simulink model "nieLiniowyModelWachadlaOdwruconego"  (R2014a)
settings: Solver=ode45  SolverMode=SingleTasking  StartTime=0.0  StopTime=100  MaxStep=0.1  MinStep=0.001  RelTol=1e-5
values from neighbouring files (symbols this model uses):
  K0 = lqr(A0,B0,Q0,R0)    [WyznaczanieParametrow.m]
  K120 = lqr(A120,B120,Q120,R120)    [WyznaczanieParametrow.m]
  K150 = acker(A150,B150,[0 3 0 0])    [WyznaczanieParametrow.m]
  K30 = lqr(A30,B30,Q30,R30)    [WyznaczanieParametrow.m]
  K90 = lqr(A90,B90,Q90,R90)    [WyznaczanieParametrow.m]
undefined symbols (not defined in the file or in its folder): K180
libraries: fuzblock x1
settings Model: CovMetricSettings=dwe  CovHtmlReporting=off  covSaveCumulativeToWorkspaceVar=off  CovSaveSingleToWorkspaceVar=off  CovExternalEMLEnable=on  CovSFcnEnable=on  Creator=Szwank  LastModifiedBy=Szwank
settings DataIOCC: LimitDataPoints=off  SaveFormat=StructureWithTime
settings DebuggingCC: MergeDetectMultiDrivingBlocksExec=error  SolverPrmCheckMsg=none  FrameProcessingCompatibilityMsg=error  SFUnexpectedBacktrackingDiag=error  SFNoUnconditionalDefaultTransitionDiag=error
settings HardwareCC: ProdBitPerPointer=64  ProdLargestAtomicFloat=Float  ProdIntDivRoundTo=Zero  ProdEndianess=LittleEndian  ProdHWDeviceType=Specified
settings ModelReferenceCC: PropagateSignalLabelsOutOfModel=on
settings GRTTargetCC: TargetLangStandard=C99 (ISO)  GeneratePreprocessorConditionals=Use local settings

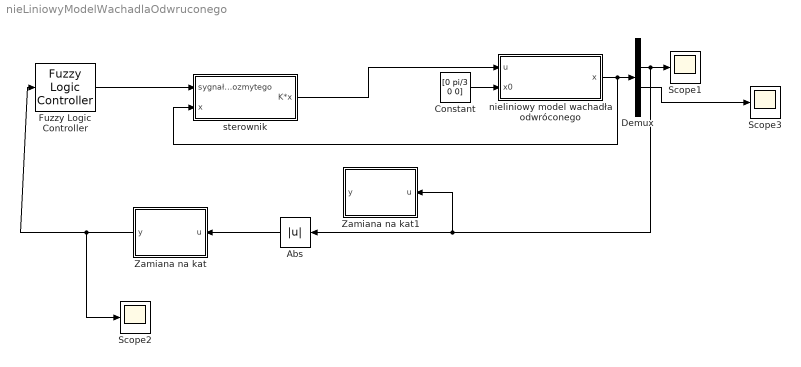
== system nieLiniowyModelWachadlaOdwruconego ==
  " nieliniowy model wachadła odwróconego" : Subsystem
  Abs : Abs
  Constant : Constant  Value=[0 pi/3 0 0]
  Demux : Demux
  Fuzzy Logic Controller : fuzblock/Fuzzy Logic  Controller  fis='modelRozmyty.fis'
  Scope1 : Scope
      settings: TimeRange=auto  MaxDataPoints=5000  SaveToWorkspace=off  YMin=-5.59281  YMax=1.78498  SampleTime=-1
  Scope2 : Scope
      settings: TimeRange=auto  MaxDataPoints=5000  SaveToWorkspace=off  YMin=-22.49983  YMax=202.49843  SampleTime=-1
  Scope3 : Scope
      settings: TimeRange=auto  MaxDataPoints=5000  SaveToWorkspace=off  SaveName=ScopeData3  YMin=-0.00269  YMax=0.0027  SampleTime=-1
  Zamiana na kat : MATLAB Function  TreatAsAtomicUnit=on
      settings: PermitHierarchicalResolution=ParametersOnly
  Zamiana na kat1 : MATLAB Function  TreatAsAtomicUnit=on
      settings: PermitHierarchicalResolution=ParametersOnly
  sterownik : Subsystem
  wires:
  Abs/1 -> Zamiana na kat/1(u)
  Zamiana na kat/1(y) -> Scope2/1, Fuzzy Logic Controller/1
  Constant/1 -> " nieliniowy model wachadła odwróconego"/2(x0)
  Demux/2 -> Zamiana na kat1/1(u), Abs/1, Scope1/1
  " nieliniowy model wachadła odwróconego"/1(x) -> sterownik/2("x "), Demux/1
  Fuzzy Logic Controller/1 -> sterownik/1(sygnał z regulatora rozmytego)
  sterownik/1(K*x) -> " nieliniowy model wachadła odwróconego"/1(u)
  Demux/3 -> Scope3/1

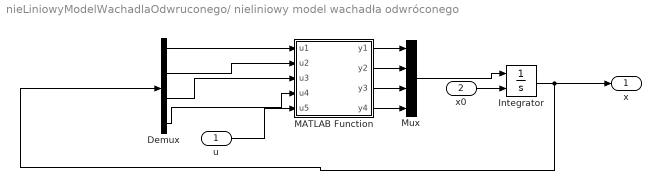
== system nieLiniowyModelWachadlaOdwruconego/ nieliniowy model wachadła odwróconego ==
  u : Inport
  x0 : Inport  Port=2
  Demux : Demux
  Integrator : Integrator  InitialConditionSource=external  InitialCondition=[0 pi/6 0 0]
  MATLAB Function : MATLAB Function  TreatAsAtomicUnit=on
      settings: PermitHierarchicalResolution=ParametersOnly
  Mux : Mux
  x : Outport
  wires:
  Mux/1 -> Integrator/1
  Demux/1 -> MATLAB Function/1(u1)
  MATLAB Function/2(y2) -> Mux/2
  Demux/4 -> MATLAB Function/4(u4)
  MATLAB Function/4(y4) -> Mux/4
  Integrator/1 -> x/1, Demux/1
  MATLAB Function/1(y1) -> Mux/1
  Demux/3 -> MATLAB Function/3(u3)
  MATLAB Function/3(y3) -> Mux/3
  Demux/2 -> MATLAB Function/2(u2)
  u/1 -> MATLAB Function/5(u5)
  x0/1 -> Integrator/2

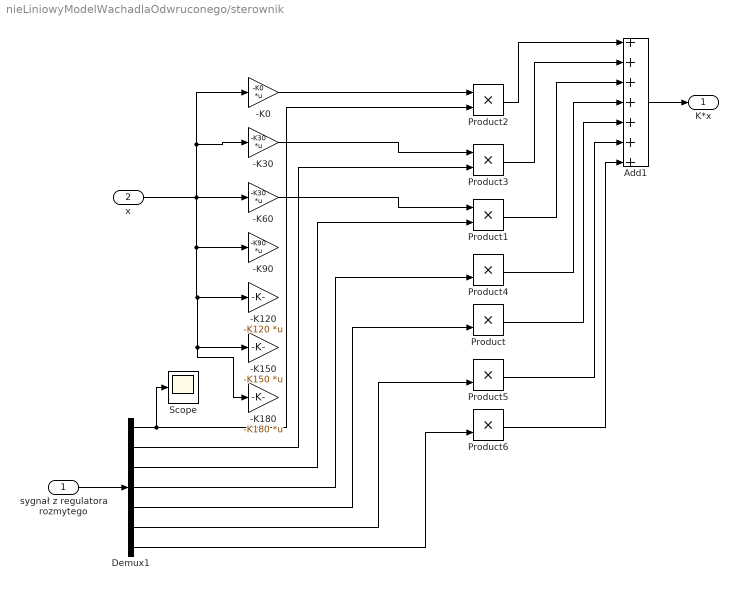
== system nieLiniowyModelWachadlaOdwruconego/sterownik ==
  sygnał z regulatora rozmytego : Inport
  "x " : Inport  Port=2
  -K0 : Gain  Gain=-K0  Multiplication=Matrix(K*u)
  "-K120 " : Gain  Gain=-K120  Multiplication=Matrix(K*u)
  "-K150 " : Gain  Gain=-K150  Multiplication=Matrix(K*u)
  -K180 : Gain  Gain=-K180  Multiplication=Matrix(K*u)
  -K30 : Gain  Gain=-K30  Multiplication=Matrix(K*u)
  -K60 : Gain  Gain=-K30  Multiplication=Matrix(K*u)
  -K90 : Gain  Gain=-K90  Multiplication=Matrix(K*u)
  Add1 : Sum  Inputs=+++++++
  Demux1 : Demux  Outputs=7
  Product{,1..6} (7 alike) : Product
  Scope : Scope
      settings: TimeRange=auto  MaxDataPoints=5000  SaveToWorkspace=off  SaveName=ScopeData2  YMin=-0.01968  YMax=1.02314  SampleTime=-1
  K*x : Outport
  wires:
  -K0/1 -> Product2/1
  sygnał z regulatora rozmytego/1 -> Demux1/1
  -K30/1 -> Product3/1
  Product3/1 -> Add1/2
  Demux1/1 -> Scope/1, Product2/2
  Product2/1 -> Add1/1
  Demux1/2 -> Product3/2
  "x "/1 -> -K180/1, "-K150 "/1, "-K120 "/1, -K90/1, -K60/1, -K30/1, -K0/1
  Add1/1 -> K*x/1
  Product1/1 -> Add1/3
  -K60/1 -> Product1/1
  Demux1/3 -> Product1/2
  Demux1/4 -> Product4/2
  Product4/1 -> Add1/4
  Demux1/5 -> Product/2
  Demux1/6 -> Product5/2
  Demux1/7 -> Product6/2
  Product/1 -> Add1/5
  Product5/1 -> Add1/6
  Product6/1 -> Add1/7

== matlab function nieLiniowyModelWachadlaOdwruconego/ nieliniowy model wachadła odwróconego/MATLAB Function ==
  data: u1 input; y1 output; u2 input; u3 input; u4 input; u5 input; y2 output; y3 output; y4 output
function [y1,y2,y3,y4] = fcn(u1,u2,u3,u4,u5)
%Dane obiektu
%% Motor
Rm = 3.3; % ohms, Motor armature resistance 
Kt = 0.0280; % N.m, Motor torque constant
Km = 0.0280; % V/(rad/s), Motor back-emf constant (same as Ktin SI units)
Jm = 9.64e-6; % kg.m2, Moment of inertia of motor rotor. 
Jeq = 1.23e-4; % kg.m2, Equivalent moment of inertia about motor shaft pivot axis.
%% Pendulum Arm:
Marm = 0.0280; % kg, Mass of the arm.
r = 0.0826; % m, Length of arm pivot to pendulum pivot.
Beq = 0.1; % N.m/(rad/s), Arm viscous damping. 
%% Pendulum Link:
Mp = 0.0270; % kg, Mass of the pendulum link and weight combined.
Lp = 0.191; % m, Total length of pendulum.
lp = 0.153; % m, Length of pendulum center of mass from pivot.
Jp = 1.20e-4; % kg.m2, Pendulum moment of inertia about its pivot axis.
Bp = 0; % N.m/(rad/s), Pendulum viscous damping.
%% Pulse-Width Modulated Amplifier:
Vmax = 24; % V, PWM amplifier maximum output voltage
PWM = 5; % A, amplifier maximum output current
Kw = 2.3; % V/V, PWM amplifier gain
%% Stałe
m = Mp;
g = 9.80665;
a = Jeq + m * r^2;
b = m * lp * r;
e = m*lp^2 + Jp;
f = m*g*lp;
c = Km*Kw/Rm;
d = (Km*Kt+Beq*Rm)/Rm;
%%

y1 = u3;
y2 = u4;
y3 = 1/(1-(b^2/(a*e))*cos(u2)^2)*(1/a)*(b*f/e*sin(u2)*cos(u2)-b*u4^2*sin(u2)+u5*c-d*u3);
y4 = 1/(1-(b^2/(a*e))*cos(u2)^2)*(1/e)*(b/a*cos(u2)*(-b*u4^2*sin(u2)+c*u5-d*u3)+f*sin(u2));

== matlab function nieLiniowyModelWachadlaOdwruconego/Zamiana na kat1 ==
  data: u input; y output
function y = fcn(u)


if(u>2*pi||u<-2*pi)
    
u=rem(u,2*pi);

end
y = u;

== matlab function nieLiniowyModelWachadlaOdwruconego/Zamiana na kat ==
  data: u input; y output
function y = fcn(u)

g=u*180/pi;
if(g>180)
    reszta=rem(g,180);
    if(rem(fix(g/180),2)==1)
        g=180-reszta;
    else
        g=reszta;
    end

end
y = g;
